simulink library "fdclib4"  (Simulink 2.09)
values from neighbouring files (symbols this model uses):
  GM1 = [cbar b    S    Ix   Iy   Iz   Jxy  Jxz  Jyz  m]    [modbuild.m]

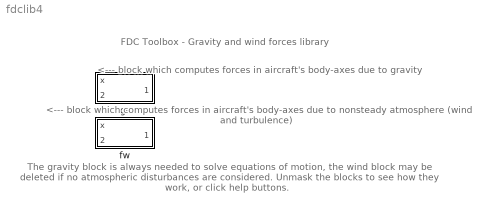
== system fdclib4 ==
  note: FDC Toolbox - Gravity and wind forces library
  note: The gravity block is always needed to solve equations of motion,
      | the wind block may be deleted if no atmospheric disturbances
      | are considered. Unmask the blocks to see how they work, or
      | click help buttons.
  note: <--- block which computes forces in
      | aircraft's body-axes due to gravity
  note: <--- block which computes forces in
      | aircraft's body-axes due to nonsteady
      | atmosphere (wind and turbulence)
  fw : Subsystem  mask(fwind){m=GM1(10)}
      mask prompts: m "Mass of the aircraft [kg]:"
      mask help: Forces due to non-steady atmosphere.
      mask Help: eval('fdchelp fwind')
      mask Display: disp('Fwind')
  gr : Subsystem  mask(Gravity){m=GM1(10)}
      mask prompts: m "Mass of the aircraft [kg]:"
      mask help: Gravity forces.
      mask Help: eval('fdchelp gravity')
      mask Display: disp('Gravity')

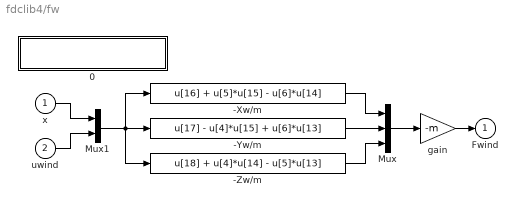
== system fdclib4/fw ==
  x : Inport  Port=1  PortWidth=-1  SampleTime=-1
  uwind : Inport  Port=2  PortWidth=-1  SampleTime=-1
  -Xw/m : Fcn  Expr=u[16] + u[5]*u[15] - u[6]*u[14]
  -Yw/m : Fcn  Expr=u[17] - u[4]*u[15] + u[6]*u[13]
  -Zw/m : Fcn  Expr=u[18] + u[4]*u[14] - u[5]*u[13]
  0 : Subsystem
      settings: OpenFcn=fdchelp fwind
      mask Display: disp('FWIND\nM.O. Rauw, Dec. 1996')
  Mux : Mux  Inputs=3
  Mux1 : Mux  Inputs=[12 6]
  gain : Gain  Gain=-m
  Fwind : Outport  Port=1  InitialOutput=0
  wires:
  -Zw/m/1 -> Mux/3
  -Xw/m/1 -> Mux/1
  -Yw/m/1 -> Mux/2
  Mux1/1 -> -Xw/m/1, -Zw/m/1, -Yw/m/1
  Mux/1 -> gain/1
  gain/1 -> Fwind/1
  x/1 -> Mux1/1
  uwind/1 -> Mux1/2

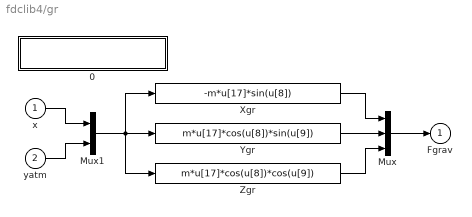
== system fdclib4/gr ==
  x : Inport  Port=1  PortWidth=-1  SampleTime=-1
  yatm : Inport  Port=2  PortWidth=-1  SampleTime=-1
  0 : Subsystem
      settings: OpenFcn=fdchelp gravity
      mask Display: disp('GRAVITY\nM.O. Rauw, October 1997')
  Mux : Mux  Inputs=3
  Mux1 : Mux  Inputs=[12 5]
  Xgr : Fcn  Expr=-m*u[17]*sin(u[8])
  Ygr : Fcn  Expr=m*u[17]*cos(u[8])*sin(u[9])
  Zgr : Fcn  Expr=m*u[17]*cos(u[8])*cos(u[9])
  Fgrav : Outport  Port=1  InitialOutput=0
  wires:
  yatm/1 -> Mux1/2
  x/1 -> Mux1/1
  Zgr/1 -> Mux/3
  Mux1/1 -> Zgr/1, Xgr/1, Ygr/1
  Mux/1 -> Fgrav/1
  Ygr/1 -> Mux/2
  Xgr/1 -> Mux/1

== system fdclib4/fw/0 ==

== system fdclib4/gr/0 ==
